simulink model "Design_a_Simulink_subsystem_to_implement_frequency_modulation"  (R2021a)
settings: Solver=VariableStepAuto  StartTime=0.0  StopTime=10.0  RelTol=1e-3
libraries: simulink x1
settings Model: Creator=Fatiha  LastModifiedBy=Fatiha

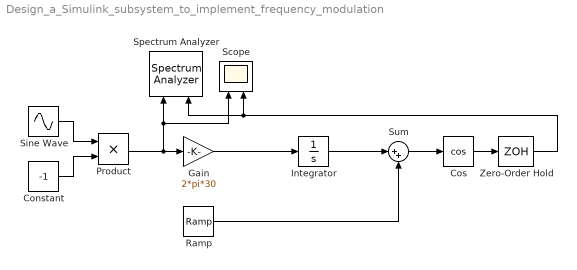
== system Design_a_Simulink_subsystem_to_implement_frequency_modulation ==
  Constant : Constant  Value=-1  SampleTime=0.0001
  Cos : Trigonometry  Operator=cos  OutputSignalType=real
  Gain : Gain  Gain=2*pi*30
  Integrator : Integrator
  Product : Product
  Ramp : simulink/Sources/Ramp  slope=2*pi*200  start=0  InitialOutput=0
  Scope : Scope  NumInputPorts=2
  Sine Wave : Sin  Frequency=2*pi*50  SampleTime=0.0001
  Spectrum Analyzer : SpectrumAnalyzer  NumInputPorts=2
  Sum : Sum  Inputs=|++
  Zero-Order Hold : ZeroOrderHold  SampleTime=-1
  wires:
  Product/1 -> Gain/1, Scope/1, Spectrum Analyzer/1
  Sine Wave/1 -> Product/1
  Constant/1 -> Product/2
  Ramp/1 -> Sum/2
  Sum/1 -> Cos/1
  Integrator/1 -> Sum/1
  Cos/1 -> Zero-Order Hold/1
  Zero-Order Hold/1 -> Scope/2, Spectrum Analyzer/2
  Gain/1 -> Integrator/1
